simulink model "RST_1ordem"  (R2015a)
settings: Solver=ode45  SolverMode=SingleTasking  StartTime=0.0  StopTime=50  RelTol=1e-3
undefined symbols (not defined in the file): A, B, Ctt, R, S, T, Ta, Tal
libraries: dspinverses x1
settings Model: CovMetricSettings=dwe  CovHtmlReporting=off  covSaveCumulativeToWorkspaceVar=off  CovSaveSingleToWorkspaceVar=off  CovExternalEMLEnable=on  Creator=tarci  LastModifiedBy=tarci
settings DataIOCC: LimitDataPoints=off  SaveFormat=Dataset
settings DebuggingCC: SFUnexpectedBacktrackingDiag=error  SFNoUnconditionalDefaultTransitionDiag=error
settings HardwareCC: ProdBitPerPointer=64  ProdLargestAtomicFloat=Float  ProdIntDivRoundTo=Zero  ProdEndianess=LittleEndian  ProdHWDeviceType=Specified
settings ModelReferenceCC: PropagateSignalLabelsOutOfModel=on
settings SFSimCC: SimUseLocalCustomCode=on
settings RTWCC: RTWUseLocalCustomCode=on
settings GRTTargetCC: TargetLangStandard=C99 (ISO)  GeneratePreprocessorConditionals=Use local settings

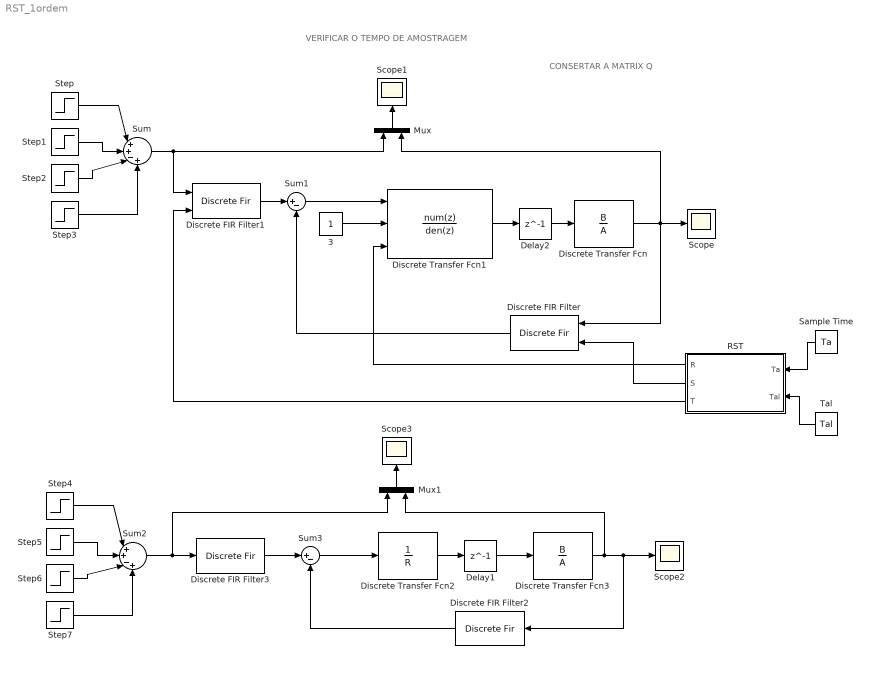
== system RST_1ordem ==
  note: CONSERTAR A MATRIX Q
  note: VERIFICAR O TEMPO DE AMOSTRAGEM
  3 : Constant
  Delay1 : Delay  DelayLength=1  InitialCondition=0  SampleTime=1
  Delay2 : Delay  DelayLength=1  InitialCondition=0  SampleTime=1
  Discrete Transfer Fcn : DiscreteTransferFcn  Numerator=B  Denominator=A  SampleTime=1
  Discrete Transfer Fcn1 : DiscreteTransferFcn  NumeratorSource=Input port  Numerator=B  DenominatorSource=Input port  Denominator=A  SampleTime=1  a0EqualsOne=on
      settings: InputPortMap=u0,p1,p3
  Discrete Transfer Fcn2 : DiscreteTransferFcn  Numerator=1  Denominator=R  SampleTime=1
  Discrete Transfer Fcn3 : DiscreteTransferFcn  Numerator=B  Denominator=A  SampleTime=1
  Discrete FIR Filter : DiscreteFir  CoefSource=Input port  SampleTime=1
  Discrete FIR Filter1 : DiscreteFir  CoefSource=Input port  SampleTime=1
  Discrete FIR Filter2 : DiscreteFir  Coefficients=S  SampleTime=1
  Discrete FIR Filter3 : DiscreteFir  Coefficients=T  SampleTime=1
  Mux : Mux  Inputs=2
  Mux1 : Mux  Inputs=2
  RST : Subsystem
  Sample Time : Constant  Value=Ta
  Scope{,1..3} (4 alike) : Scope
      Scope settings: TimeRange=auto  MaxDataPoints=5000  SaveToWorkspace=off  YMin=-0.36144  YMax=3.25296  SampleTime=-1
      Scope1 settings: TimeRange=auto  MaxDataPoints=5000  SaveToWorkspace=off  SaveName=ScopeData2  YMin=-0.5  YMax=4.5  SampleTime=-1
      Scope2 settings: TimeRange=auto  MaxDataPoints=5000  SaveToWorkspace=off  SaveName=ScopeData3  YMin=-0.73435  YMax=6.60919  SampleTime=-1
      Scope3 settings: TimeRange=auto  MaxDataPoints=5000  SaveToWorkspace=off  SaveName=ScopeData  YMin=-0.5  YMax=4.5  SampleTime=-1
  Step : Step  SampleTime=0
  Step1 : Step  Time=10  After=3  SampleTime=0
  Step2 : Step  Time=20  After=2  SampleTime=0
  Step3 : Step  Time=30  SampleTime=0
  Step4 : Step  SampleTime=0
  Step5 : Step  Time=10  After=3  SampleTime=0
  Step6 : Step  Time=20  After=2  SampleTime=0
  Step7 : Step  Time=30  SampleTime=0
  Sum : Sum  Inputs=|++-+
  Sum1 : Sum  Inputs=|+-
  Sum2 : Sum  Inputs=|++-+
  Sum3 : Sum  Inputs=|+-
  Tal : Constant  Value=Tal
  wires:
  Discrete Transfer Fcn/1 -> Discrete FIR Filter/1, Scope/1, Mux/2
  Step/1 -> Sum/1
  Mux1/1 -> Scope3/1
  Tal/1 -> RST/2(Tal)
  Discrete FIR Filter/1 -> Sum1/2
  Discrete Transfer Fcn2/1 -> Delay1/1
  Sum1/1 -> Discrete Transfer Fcn1/1
  Discrete FIR Filter3/1 -> Sum3/1
  Step4/1 -> Sum2/1
  Discrete FIR Filter2/1 -> Sum3/2
  Step5/1 -> Sum2/2
  Discrete Transfer Fcn3/1 -> Scope2/1, Discrete FIR Filter2/1, Mux1/2
  Sum2/1 -> Mux1/1, Discrete FIR Filter3/1
  Step6/1 -> Sum2/3
  Discrete Transfer Fcn1/1 -> Delay2/1
  Step2/1 -> Sum/3
  Sum3/1 -> Discrete Transfer Fcn2/1
  Sum/1 -> Discrete FIR Filter1/1, Mux/1
  3/1 -> Discrete Transfer Fcn1/2
  Sample Time/1 -> RST/1(Ta)
  Discrete FIR Filter1/1 -> Sum1/1
  Step7/1 -> Sum2/4
  Mux/1 -> Scope1/1
  Delay1/1 -> Discrete Transfer Fcn3/1
  Step3/1 -> Sum/4
  Step1/1 -> Sum/2
  Delay2/1 -> Discrete Transfer Fcn/1
  RST/1(R) -> Discrete Transfer Fcn1/3
  RST/2(S) -> Discrete FIR Filter/2
  RST/3(T) -> Discrete FIR Filter1/2

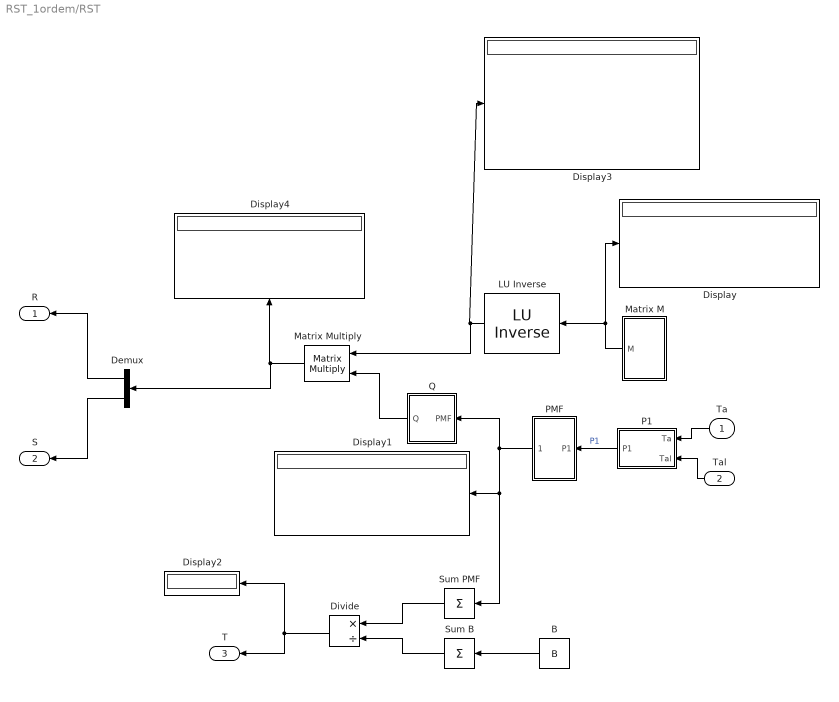
== system RST_1ordem/RST ==
  Ta : Inport
  Tal : Inport  Port=2
  " LU Inverse" : dspinverses/ LU Inverse
  B : Constant  Value=B
  Demux : Demux  Outputs=2
  Display{,1..4} (5 alike) : Display
  Divide : Product  Inputs=*/
  Matrix M : Subsystem
  Matrix Multiply : Product  Multiplication=Matrix(*)
  P1 : Subsystem
  PMF : Subsystem
  Q : Subsystem
  Sum B : Sum  Inputs=+
  Sum PMF : Sum  Inputs=+
  R : Outport
  S : Outport  Port=2
  T : Outport  Port=3
  wires:
  Tal/1 -> P1/2(Tal)
  Ta/1 -> P1/1(Ta)
  Matrix M/1(M) -> " LU Inverse"/1, Display/1
  P1/1(P1) -> PMF/1(P1)  "P1"
  PMF/1(PMF) -> Q/1(PMF), Sum PMF/1, Display1/1
  Sum PMF/1 -> Divide/1
  B/1 -> Sum B/1
  Sum B/1 -> Divide/2
  Divide/1 -> T/1, Display2/1
  " LU Inverse"/1 -> Matrix Multiply/1, Display3/1
  Matrix Multiply/1 -> Demux/1, Display4/1
  Q/1(Q) -> Matrix Multiply/2
  Demux/1 -> R/1
  Demux/2 -> S/1

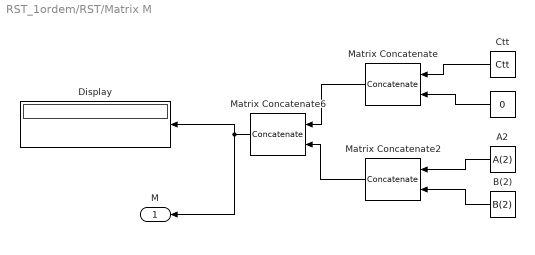
== system RST_1ordem/RST/Matrix M ==
  " " : Constant  Value=0
  " B(2)" : Constant  Value=B(2)
  A2 : Constant  Value=A(2)
  Ctt : Constant  Value=Ctt
  Display : Display
  Matrix Concatenate : Concatenate  Mode=Multidimensional array  ConcatenateDimension=2
  Matrix Concatenate2 : Concatenate  Mode=Multidimensional array  ConcatenateDimension=2
  Matrix Concatenate6 : Concatenate  Mode=Multidimensional array
  M : Outport
  wires:
  " "/1 -> Matrix Concatenate/2
  Ctt/1 -> Matrix Concatenate/1
  " B(2)"/1 -> Matrix Concatenate2/2
  Matrix Concatenate/1 -> Matrix Concatenate6/1
  Matrix Concatenate2/1 -> Matrix Concatenate6/2
  A2/1 -> Matrix Concatenate2/1
  Matrix Concatenate6/1 -> M/1, Display/1

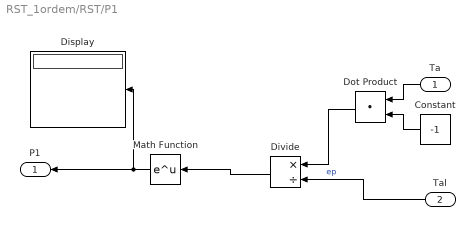
== system RST_1ordem/RST/P1 ==
  Ta : Inport
  Tal : Inport  Port=2
  Constant : Constant  Value=-1
  Display : Display
  Divide : Product  Inputs=*/
  Dot Product : DotProduct  InputSameDT=on  OutDataTypeStr=Inherit: Inherit via internal rule
  Math Function : Math  SaturateOnIntegerOverflow=on
  P1 : Outport
  wires:
  Ta/1 -> Dot Product/1
  Dot Product/1 -> Divide/1
  Tal/1 -> Divide/2  "ep"
  Divide/1 -> Math Function/1
  Math Function/1 -> Display/1, P1/1
  Constant/1 -> Dot Product/2

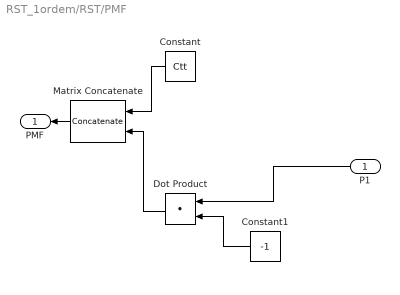
== system RST_1ordem/RST/PMF ==
  P1 : Inport
  Constant : Constant  Value=Ctt
  Constant1 : Constant  Value=-1
  Dot Product : DotProduct  InputSameDT=on  OutDataTypeStr=Inherit: Inherit via internal rule
  Matrix Concatenate : Concatenate  Mode=Multidimensional array  ConcatenateDimension=2
  PMF : Outport
  wires:
  Constant1/1 -> Dot Product/2
  Constant/1 -> Matrix Concatenate/1
  Dot Product/1 -> Matrix Concatenate/2
  P1/1 -> Dot Product/1
  Matrix Concatenate/1 -> PMF/1

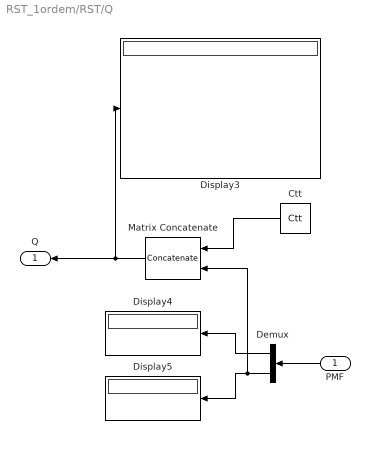
== system RST_1ordem/RST/Q ==
  PMF : Inport
  Ctt : Constant  Value=Ctt
  Demux : Demux  Outputs=2
  Display3 : Display
  Display4 : Display
  Display5 : Display
  Matrix Concatenate : Concatenate  Mode=Multidimensional array
  Q : Outport
  wires:
  Demux/1 -> Display4/1
  PMF/1 -> Demux/1
  Demux/2 -> Matrix Concatenate/2, Display5/1
  Ctt/1 -> Matrix Concatenate/1
  Matrix Concatenate/1 -> Q/1, Display3/1
